simulink model "Lab3_ME13"  (R2021b)
settings: Solver=ode1  StartTime=0.0  StopTime=100  FixedStep=Ts  RelTol=1e-3
InitFcn:
  | Ts=1e-3;
  | Tfi=10e-3;
  | P_struja=1.65;
  | I_struja=65;
  | Tfb=10e-3;
  | Ce = 0.0134*8000/146;
undefined symbols (not defined in the file or in its folder): rtblkgui
libraries: simulink x4, slpidlib x1
settings Model: SimulationMode=external  ExtModeTrigDuration=10001  Creator=Labos1  LastModifiedBy=Melab1Guest
settings SolverCC: AlgebraicLoopSolver=TrustRegion
settings DataIOCC: MaxDataPoints=10001  ReturnWorkspaceOutputs=off
settings OptimizationCC: LifeSpan=inf
settings DebuggingCC: SFExecutionAtInitializationDiag=none  SFMachineParentedDataDiag=warning  ArithmeticOperatorsInVariantConditions=warning
settings SFSimCC: SimUseLocalCustomCode=off  CustomCodeUndefinedFunction=UseInterfaceOnly
settings RTWCC: Description=Simulink Desktop Real-Time  SystemTargetFile=sldrt.tlc  TemplateMakefile=sldrt.tmf  RTWUseLocalCustomCode=off  RTWCompilerOptimization=on
settings CodeAppCC: MaxIdLength=95  StateflowObjectComments=on
settings SimulinkDesktopRealTimeCC: TargetPreCompLibLocation=C:\Program Files\MATLAB\R2021b\toolbox\sldrt\lib\win64  SupportVariableSizeSignals=off

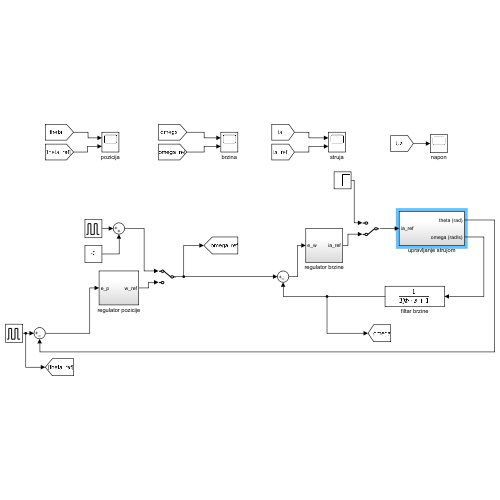
[thumbnail: Simulink's stored preview of the top-level diagram]
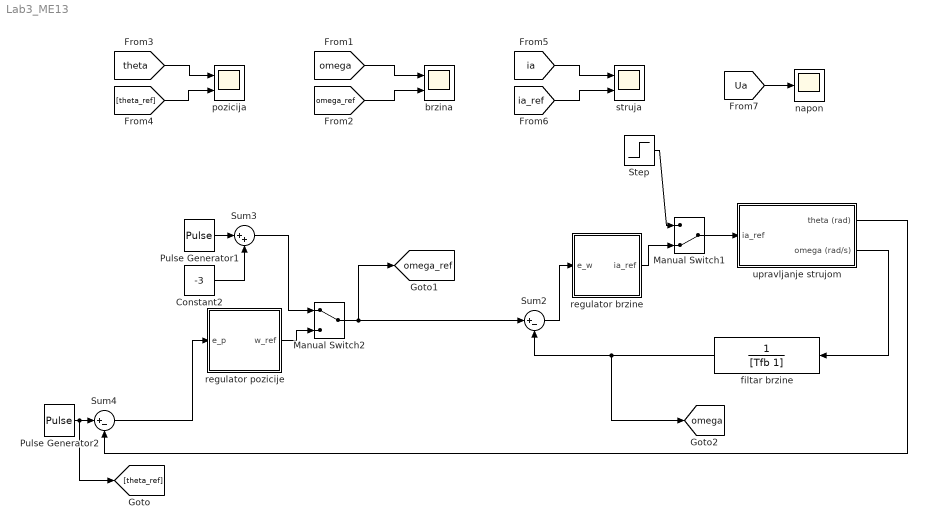
== system Lab3_ME13 ==
  Constant2 : Constant  Value=-3
  Manual Switch1 : ManualSwitch  CurrentSetting=0
  Manual Switch2 : ManualSwitch
  Pulse Generator1 : DiscretePulseGenerator  PulseType=Time based  Amplitude=6  Period=10  PulseWidth=50
  Pulse Generator2 : DiscretePulseGenerator  PulseType=Time based  Period=60  PulseWidth=50
  Step : Step  After=0  SampleTime=0
  Sum2 : Sum  Inputs=|+-
  Sum3 : Sum  Inputs=|++
  Sum4 : Sum  Inputs=|+-
  brzina : Scope  NumInputPorts=2
  filtar brzine : TransferFcn  Denominator=[Tfb 1]
  napon : Scope
  pozicija : Scope  NumInputPorts=2
  regulator brzine : Subsystem
  regulator pozicije : Subsystem
  struja : Scope  NumInputPorts=2
  upravljanje strujom : Subsystem
  tag scope: omega=global, omega_ref=global
  wires:
  Pulse Generator1/1 -> Sum3/1
  Constant2/1 -> Sum3/2
  Sum3/1 -> Manual Switch2/1
  [omega] -> brzina/1
  [omega_ref] -> brzina/2
  Manual Switch1/1 -> upravljanje strujom/1(ia_ref)
  Sum2/1 -> regulator brzine/1(e_w)
  regulator brzine/1(ia_ref) -> Manual Switch1/2
  upravljanje strujom/2(omega (rad/s)) -> filtar brzine/1
  [theta_ref] -> pozicija/2
  [theta] -> pozicija/1
  [ia_ref] -> struja/2
  [ia] -> struja/1
  [Ua] -> napon/1
  upravljanje strujom/1(theta (rad)) -> Sum4/2
  Pulse Generator2/1 -> [theta_ref], Sum4/1
  Manual Switch2/1 -> Sum2/1, [omega_ref]
  regulator pozicije/1(w_ref) -> Manual Switch2/2
  filtar brzine/1 -> [omega], Sum2/2
  Sum4/1 -> regulator pozicije/1(e_p)
  Step/1 -> Manual Switch1/1

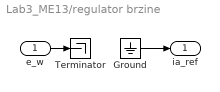
== system Lab3_ME13/regulator brzine ==
  e_w : Inport
  Ground : Ground
  Terminator : Terminator
  ia_ref : Outport
  wires:
  e_w/1 -> Terminator/1
  Ground/1 -> ia_ref/1

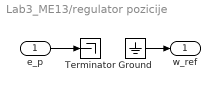
== system Lab3_ME13/regulator pozicije ==
  e_p : Inport
  Ground : Ground
  Terminator : Terminator
  w_ref : Outport
  wires:
  e_p/1 -> Terminator/1
  Ground/1 -> w_ref/1

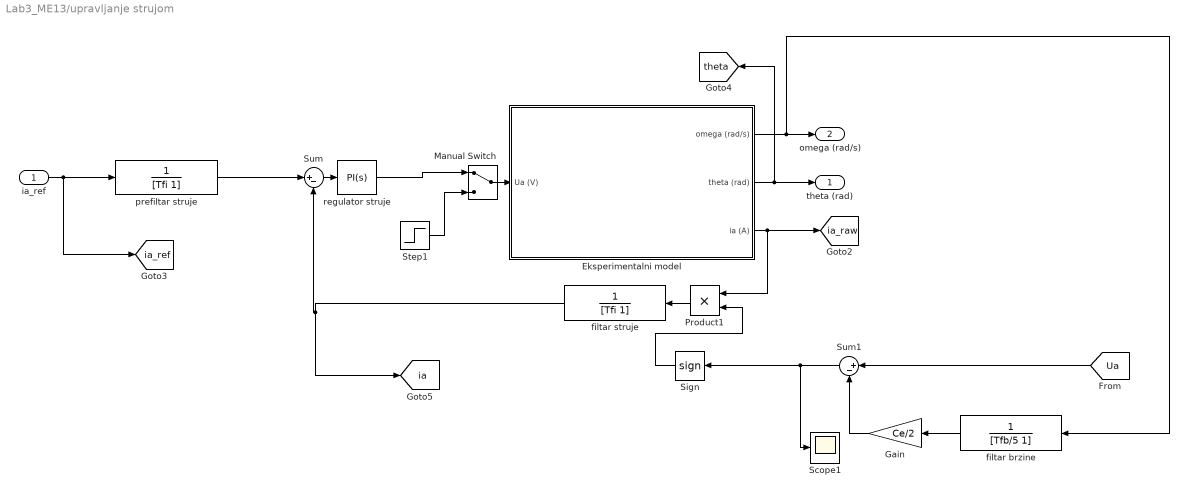
== system Lab3_ME13/upravljanje strujom ==
  ia_ref : Inport
  Eksperimentalni model : Subsystem  mask{R6=383, motorRes=2849.3, Ts=Ts}
      mask init:
      | currentBlock = gcb;
      | %% Closing all the ports:
      | Port = '';
      | FullPort = '';
      | if ~isempty(instrfind)
      |     fclose(instrfind);
      |     delete(instrfind);
      | end
      | %% Find all the COM ports in a computer
      | s1 = instrhwinfo('serial');
      | coms = s1.AvailableSerialPorts;
      | key = 'HKEY_LOCAL_MACHINE\SYSTEM\CurrentControlSet\Enum\USB\';
      | % Find all installed USB devices entries and clean up the output
      | [~, vals] = dos(['REG QUERY ' key ' /s /f "FriendlyName" /t "REG_SZ"']);
      | vals = textscan(vals,'%s','delimiter','\t');
      | vals = cat(1,vals{:});
      | out = 0;
      | % Find all friendly name property entries
      | for i = 1:numel(vals)
      |     if strcmp(vals{i}(1:min(12,end)),'FriendlyName')
      |         if ~iscell(out)
      |             out = vals(i);
      |         else
      |             out{end+1} = vals{i};
      |         end
      |     end
      | end
      | % Compare friendly name entries with connected ports and generate output
      | devs = cell(numel(coms),2);
      | for i = 1:numel(coms)
      |   match = strfind(out,[coms{i},')']);
      |   ind = 0;
      |   for j = 1:numel(match)
      |       if ~isempty(match{j})
      |           ind = j;
      |       end
      |   end
      |   if ind ~= 0
      |       com = str2double(coms{i}(4:end));
      | % Trim the trailing ' (COM##)' from the friendly name - works on ports from 1 to 99
      |       if com > 9
      |           length = 8;
      |       else
      |           length = 7;
      |       end
      |       devs{i,1} = out{ind}(27:end-length);
      |       devs{i,2} = com;
      |   end
      | end
      | % Find USB device
      | for i = size(devs,1)
      |     if strfind(devs{i,1},'USB Serial Device')
      |         ind = i;
      |     end
      | end
      | if ~ind
      |     Port = [];
      | else
      |     port = coms(ind);
      |     Port = port{1};
      | end
      | if (isempty(Port))
      |  %   msgbox('Barbell lab board not found, make sure it is connected, FTDI driver is installed and try again')
      | else
      |     %% Set Packet Input and Packet Output parameters
      |     po = strcat(currentBlock,'/Packet Output1');
      |     pinput = strcat(currentBlock,'/Packet Input1');
      |     %%
      |     set_param(po, 'LinkStatus','inactive');
      |     set_param(pinput, 'LinkStatus','inactive');
      |     %%
      |     p = Simulink.Mask.get(po);
      |     a = p.Parameters(6);
      |     FullPort = Port;
      |     Port = replace(Port,'COM','');
      |     if isempty(Port)
      |         Port = a.Value
      |     end
      |     %%
      | 
      |     a.set('Value',Port);
      |     %%
      |     %%
      |     %%
      |     p1 = Simulink.Mask.get(pinput);
      |     a1 = p1.Parameters(6);
      |     a1.set('Value',Port);
      | 
      | end
      mask Display:
      | ud = get_param(gcb,'UserData');
      | image(ud.x);
  Gain : Gain  Gain=Ce/2
  Manual Switch : ManualSwitch
  Product1 : Product
  Scope1 : Scope
  Sign : Signum
  Step1 : Step  After=6  SampleTime=0
  Sum : Sum  Inputs=|+-
  Sum1 : Sum  Inputs=|+-
  filtar brzine : TransferFcn  Denominator=[Tfb/5 1]
  filtar struje : TransferFcn  Denominator=[Tfi 1]
  prefiltar struje : TransferFcn  Denominator=[Tfi 1]
  regulator struje : slpidlib/PID Controller  Controller=PI  Form=Parallel  TimeDomain=Continuous-time  UseExternalTs=off  SampleTime=-1  IntegratorMethod=Forward Euler  FilterMethod=Forward Euler  ControllerParametersSource=internal  P=P_struja  I=I_struja  D=0  UseFilter=on  N=100  TunerSelectOption=Transfer Function Based (PID Tuner App)  InitialConditionSource=internal  InitialConditionForIntegrator=0  InitialConditionForFilter=0  DifferentiatorICPrevScaledInput=0  ExternalReset=none  TrackingMode=off  Kt=1  LimitOutput=on  SatLimitsSource=internal  UpperSaturationLimit=12  LowerSaturationLimit=-12  LinearizeAsGain=on  AntiWindupMode=clamping  Kb=100  POutMin=[]  POutMax=[]  IOutMin=[]  IOutMax=[]  DOutMin=[]  DOutMax=[]  NOutMin=[]  NOutMax=[]  SumOutMin=[]  SumOutMax=[]  SaturationOutMin=[]  SaturationOutMax=[]  PParamMin=[]  PParamMax=[]  IParamMin=[]  IParamMax=[]  DParamMin=[]  DParamMax=[]  NParamMin=[]  NParamMax=[]  KbParamMin=[]  KbParamMax=[]  KtParamMin=[]  KtParamMax=[]  KbOutMin=[]  KbOutMax=[]  KtOutMin=[]  KtOutMax=[]  IntegratorOutMin=[]  IntegratorOutMax=[]  FilterOutMin=[]  FilterOutMax=[]  SumI1OutMin=[]  SumI1OutMax=[]  SumI2OutMin=[]  SumI2OutMax=[]  SumI3OutMin=[]  SumI3OutMax=[]  SumI4OutMin=[]  SumI4OutMax=[]  SumDOutMin=[]  SumDOutMax=[]  DifferentiatorOutMin=[]  DifferentiatorOutMax=[]  FilterDiffOutCoefMin=[]  FilterDiffOutCoefMax=[]  ReciprocalOutMin=[]  ReciprocalOutMax=[]  SumDenOutMin=[]  SumDenOutMax=[]  SumNumOutMin=[]  SumNumOutMax=[]  DivideOutMin=[]  DivideOutMax=[]  UdiffTsProdOutMin=[]  UdiffTsProdOutMax=[]  NTsProdOutMin=[]  NTsProdOutMax=[]  UintegralTsProdOutMin=[]  UintegralTsProdOutMax=[]  UngainTsProdOutMin=[]  UngainTsProdOutMax=[]  IntegratorContinuousStateAttributes=''  IntegratorStateMustResolveToSignalObject=off  IntegratorRTWStateStorageClass=Auto  FilterContinuousStateAttributes=''  FilterStateMustResolveToSignalObject=off  FilterRTWStateStorageClass=Auto  ParallelPVariant=InternalParameters  IdealPVariant=Disabled  IVariant=InternalParameters  DVariant=Disabled  IntegratorVariant=Continuous  SatVariant=Enabled  AWVariant=ContClampingParallel  PCopyVariant=Disabled  TRVariant=Disabled  FdbkBlocksVariant=Forward  IdealPFdbkVariant=Disabled  SatFdbkVariant=Disabled  DerivativeFilterVariant=Disabled  NVariant=Disabled  NCopyVariant=Disabled_SignalSpec  FilterICVariant=Disabled  IntegratorICVariant=InternalICs  ExternalResetVariant=Disabled  TRSumVariant=Passthrough  SumFdbkVariant=Disabled  SumVariant=Sum_PI  TsampFilterVariant=InternalTs  TsampNgainVariant=Passthrough  TsampIntegralVariant=Passthrough  ExternalSaturationOutDataTypeStr=Inherit: Same as second input
  theta (rad) : Outport
  omega (rad/s) : Outport  Port=2
  tag scope: ia=global, ia_raw=global, ia_ref=global, theta=global
  wires:
  prefiltar struje/1 -> Sum/1
  Sum/1 -> regulator struje/1
  Manual Switch/1 -> Eksperimentalni model/1(Ua (V))
  Step1/1 -> Manual Switch/2
  Eksperimentalni model/2(theta (rad)) -> [theta], theta (rad)/1
  [Ua] -> Sum1/1
  Gain/1 -> Sum1/2
  Sum1/1 -> Scope1/1, Sign/1
  Eksperimentalni model/1(omega (rad/s)) -> filtar brzine/1, omega (rad/s)/1
  Eksperimentalni model/3(ia (A)) -> Product1/1, [ia_raw]
  filtar brzine/1 -> Gain/1
  filtar struje/1 -> [ia], Sum/2
  Sign/1 -> Product1/2
  Product1/1 -> filtar struje/1
  regulator struje/1 -> Manual Switch/1
  ia_ref/1 -> [ia_ref], prefiltar struje/1

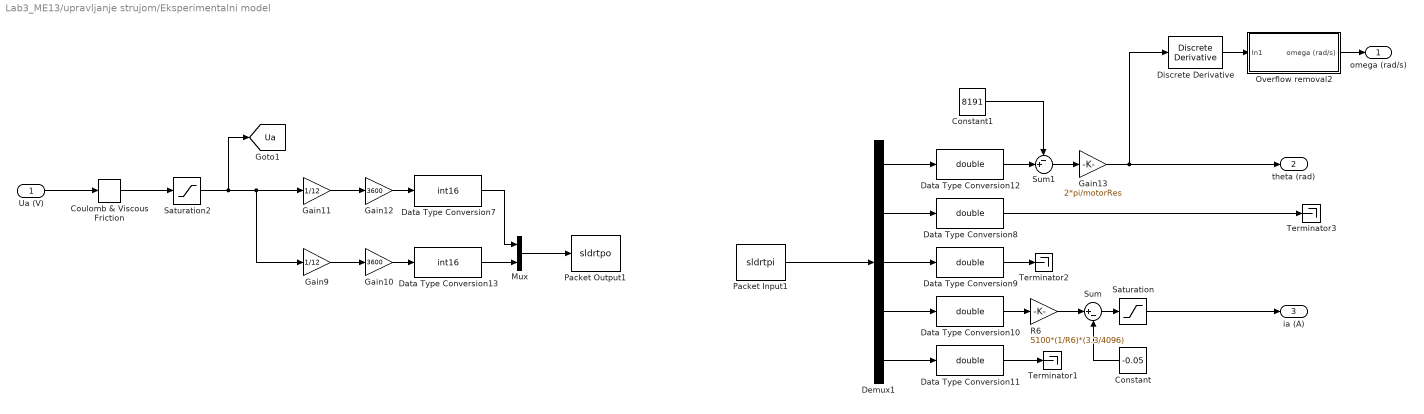
== system Lab3_ME13/upravljanje strujom/Eksperimentalni model ==
  Ua (V) : Inport
  Constant : Constant  Value=-0.05
  Constant1 : Constant  Value=8191
  Coulomb & Viscous Friction : simulink/Discontinuities/Coulomb & Viscous Friction  offset=1.5  gain=1
  Data Type Conversion{8..12} (5 alike) : DataTypeConversion  OutDataTypeStr=double
  Data Type Conversion13 : DataTypeConversion  OutDataTypeStr=int16
  Data Type Conversion7 : DataTypeConversion  OutDataTypeStr=int16
  Demux1 : Demux  Outputs=5
  Discrete Derivative : simulink/Discrete/Discrete Derivative  gainval=1.0  ICPrevScaledInput=0.0  OutMin=[]  OutMax=[]  OutDataType=fixdt(1, 16)  OutScaling=2^-10  DoSatur=off
  Gain10 : Gain  Gain=3600
  Gain11 : Gain  Gain=1/12
  Gain12 : Gain  Gain=3600
  Gain13 : Gain  Gain=2*pi/motorRes  OutDataTypeStr=double
  Gain9 : Gain  Gain=1/12
  Mux : Mux  Inputs=2
  Overflow removal2 : Subsystem
  Packet Input1 : S-Function  AncestorBlock=sldrtlib/Packet Input  LoadFcn=rtblkgui('Load')  StartFcn=rtblkgui('Start',1)  StopFcn=rtblkgui('Start',0)  FunctionName=sldrtpi  Parameters=SampleTime,MaxMissedTicks,ShowMissedTicks,YieldWhenWaiting,DrvName,DrvAddress,DrvOptions,PacketSize,DataTypes,ShowReady,ShowError,PacketID,ByteOrder,ShowTimestamp  SFunctionDeploymentMode=off  EnableBusSupport=off  mask(Simulink Desktop Real-Time Packet Input){SampleTime=Ts, MaxMissedTicks=10, ShowMissedTicks=off, YieldWhenWaiting=off, DrvName=Standard_Devices/Serial_Port, DrvAddress=3, DrvOptions=[115200 8 0 0 0 0 0 0], PacketSize=5*2, DataTypes='5*int16', ShowReady=off, ShowError=off, PacketID=1, ByteOrder=1, ShowTimestamp=off}
      mask prompts: SampleTime "sldrt:sldrtlib:ParamSampleTime"; MaxMissedTicks "sldrt:sldrtlib:ParamMaxMissedTicks"; ShowMissedTicks "sldrt:sldrtlib:ParamShowMissedTicks"; YieldWhenWaiting "sldrt:sldrtlib:ParamYieldWhenWaiting"; DrvName "sldrt:sldrtlib:ParamDriverName"; DrvAddress "sldrt:sldrtlib:ParamDriverAddress"; DrvOptions "sldrt:sldrtlib:ParamDriverOptions"; PacketSize "sldrt:sldrtlib:ParamInputPacketSize"; DataTypes "sldrt:sldrtlib:ParamPacketInputDataTypes"; ShowReady "sldrt:sldrtlib:ParamShowDataReady"; ShowError "sldrt:sldrtlib:ParamShowDataError"; PacketID "sldrt:sldrtlib:ParamPacketIdentifier"; ByteOrder "sldrt:sldrtlib:ParamPacketInputByteOrder"; ShowTimestamp "sldrt:sldrtlib:ParamShowPacketTimestamp"
      mask help: sldrt:sldrtlib:DescPacketInput
      settings: AttributesFormatString=Serial Port [3]  ModelCloseFcn=close(findall(0, 'Type', 'figure', 'Tag', 'SLDRT_RTBLKGUI', 'UserData', gcbh))  OpenFcn=rtblkgui('Open','PI')  ParentCloseFcn=eval(get_param(gcbh, 'ModelCloseFcn'))
      mask Help: helpview(fullfile(docroot, 'toolbox', 'sldrt', 'helptargets.map'), 'rtw_packet_in')
      mask Display: disp('Packet\nInput')
  Packet Output1 : S-Function  AncestorBlock=sldrtlib/Packet Output  LoadFcn=rtblkgui('Load')  StartFcn=rtblkgui('Start',1)  StopFcn=rtblkgui('Start',0)  FunctionName=sldrtpo  Parameters=SampleTime,MaxMissedTicks,ShowMissedTicks,YieldWhenWaiting,DrvName,DrvAddress,DrvOptions,PacketSize,DataTypes,ShowReady,ShowError,PacketID,ByteOrder,InitialValue,FinalValue  SFunctionDeploymentMode=off  EnableBusSupport=off  mask(Simulink Desktop Real-Time Packet Output){SampleTime=Ts, MaxMissedTicks=10, ShowMissedTicks=off, YieldWhenWaiting=off, DrvName=Standard_Devices/Serial_Port, DrvAddress=3, DrvOptions=[115200 8 0 0 0 0 0 0], PacketSize=4, DataTypes='2*int16', ShowReady=off, ShowError=off, PacketID=1, ByteOrder=1, InitialValue=[32767 2], FinalValue=[0 0]}
      mask prompts: SampleTime "sldrt:sldrtlib:ParamSampleTime"; MaxMissedTicks "sldrt:sldrtlib:ParamMaxMissedTicks"; ShowMissedTicks "sldrt:sldrtlib:ParamShowMissedTicks"; YieldWhenWaiting "sldrt:sldrtlib:ParamYieldWhenWaiting"; DrvName "sldrt:sldrtlib:ParamDriverName"; DrvAddress "sldrt:sldrtlib:ParamDriverAddress"; DrvOptions "sldrt:sldrtlib:ParamDriverOptions"; PacketSize "sldrt:sldrtlib:ParamOutputPacketSize"; DataTypes "sldrt:sldrtlib:ParamPacketOutputDataTypes"; ShowReady "sldrt:sldrtlib:ParamShowDataReady"; ShowError "sldrt:sldrtlib:ParamShowDataError"; PacketID "sldrt:sldrtlib:ParamPacketIdentifier"; ByteOrder "sldrt:sldrtlib:ParamPacketOutputByteOrder"; InitialValue "sldrt:sldrtlib:ParamInitialValue"; FinalValue "sldrt:sldrtlib:ParamFinalValue"
      mask help: sldrt:sldrtlib:DescPacketOutput
      settings: AttributesFormatString=Serial Port [3]  ModelCloseFcn=close(findall(0, 'Type', 'figure', 'Tag', 'SLDRT_RTBLKGUI', 'UserData', gcbh))  OpenFcn=rtblkgui('Open','PO')  ParentCloseFcn=eval(get_param(gcbh, 'ModelCloseFcn'))
      mask Help: helpview(fullfile(docroot, 'toolbox', 'sldrt', 'helptargets.map'), 'rtw_packet_out')
      mask Display: disp('Packet\nOutput')
  R6 : Gain  Gain=5100*(1/R6)*(3.3/4096)
  Saturation : Saturate  UpperLimit=10  LowerLimit=0
  Saturation2 : Saturate  UpperLimit=9  LowerLimit=-9
  Sum : Sum  Inputs=|+-
  Sum1 : Sum  Inputs=-+|
  Terminator1 : Terminator
  Terminator2 : Terminator
  Terminator3 : Terminator
  omega (rad/s) : Outport  VectorParamsAs1DForOutWhenUnconnected=off
  theta (rad) : Outport  Port=2
  ia (A) : Outport  Port=3
  tag scope: Ua=global
  wires:
  Gain12/1 -> Data Type Conversion7/1
  Gain11/1 -> Gain12/1
  Gain10/1 -> Data Type Conversion13/1
  Gain9/1 -> Gain10/1
  Demux1/1 -> Data Type Conversion12/1
  Demux1/2 -> Data Type Conversion8/1
  Demux1/3 -> Data Type Conversion9/1
  Demux1/4 -> Data Type Conversion10/1
  Demux1/5 -> Data Type Conversion11/1
  Data Type Conversion7/1 -> Mux/1
  Data Type Conversion13/1 -> Mux/2
  Data Type Conversion8/1 -> Terminator3/1
  Gain13/1 -> theta (rad)/1, Discrete Derivative/1
  Discrete Derivative/1 -> Overflow removal2/1(In1)
  Overflow removal2/1(omega (rad/s)) -> omega (rad/s)/1
  Mux/1 -> Packet Output1/1
  Data Type Conversion11/1 -> Terminator1/1
  Data Type Conversion10/1 -> R6/1
  Data Type Conversion9/1 -> Terminator2/1
  Packet Input1/1 -> Demux1/1
  R6/1 -> Sum/1
  Sum/1 -> Saturation/1
  Constant/1 -> Sum/2
  Saturation/1 -> ia (A)/1
  Saturation2/1 -> [Ua], Gain9/1, Gain11/1
  Coulomb & Viscous Friction/1 -> Saturation2/1
  Ua (V)/1 -> Coulomb & Viscous Friction/1
  Sum1/1 -> Gain13/1
  Data Type Conversion12/1 -> Sum1/2
  Constant1/1 -> Sum1/1

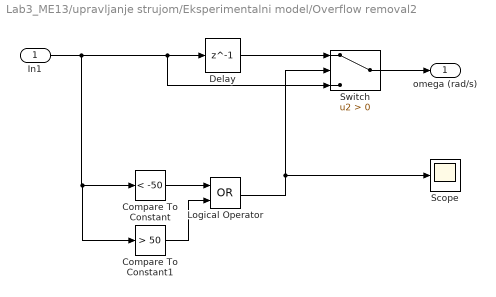
== system Lab3_ME13/upravljanje strujom/Eksperimentalni model/Overflow removal2 ==
  In1 : Inport
  Compare To Constant : simulink/Logic and Bit Operations/Compare To Constant  relop=<  const=-50  OutDataTypeStr=boolean
  Compare To Constant1 : simulink/Logic and Bit Operations/Compare To Constant  relop=>  const=50  OutDataTypeStr=boolean
  Delay : Delay  DelayLength=1  InitialCondition=0  UseCircularBuffer=on
  Logical Operator : Logic  Operator=OR  AllPortsSameDT=off  OutDataTypeStr=boolean
  Scope : Scope
  Switch : Switch  Criteria=u2 > Threshold
  omega (rad/s) : Outport  VectorParamsAs1DForOutWhenUnconnected=off
  wires:
  In1/1 -> Switch/3, Delay/1, Compare To Constant1/1, Compare To Constant/1
  Compare To Constant/1 -> Logical Operator/1
  Compare To Constant1/1 -> Logical Operator/2
  Delay/1 -> Switch/1
  Switch/1 -> omega (rad/s)/1
  Logical Operator/1 -> Scope/1, Switch/2
